simulink model "mfordmodel_v1"  (R2023a)
settings: Solver=ode45  StartTime=0.0  StopTime=10.0  RelTol=1e-3  EnableMultiTasking=on
undefined symbols (not defined in the file): ABV_RATIO_SW, AC_OFF_DLY, ACLOD, AUTO_TRNS_SW, BRAKE_DNDT_X, BZZRPM, BZZRPM_ALT, BZZTM, BZZTM_ALT, CMD_LITOFF, CMD_STABLE, CO_ST_ECT__A, COOL_BASE, DAS_BKDLY_A, DAS_CNT, DAS_CTDLY, DAS_LC_SW__A, DASCLP_5INH, DASCTL, DASMHYST, DASMPH, DEBYCP, DES_BASE, DPNEU_MUL, DSDRPM_DN_TC, DSDRPM_OFF, DSDRPM_UP_TC, EDF_DELAY, EDFHP, ETC_CL_TP, ETC_HP, GR_CM_CREEP, HCAM_ACT_CLP, HEDFHP, HEDFRPM, HICAM_PS, IAC_CAL_SW, IAC_ER_TM1, IAC_ER_TM2, IAC_ER_TM4, IAC_HI_LIM__A, IAC_ISFL_OBD, IAC_KAM_SW, IAC_LO_LIM__A, IAC_MON_TM, IAC_OT_REQ, IAC_RUN_TM, IAC_TP_OBD, IAC_TR_DAS, IAC_TST_DC, ID_DAS__A, ID_NOVS__A, IDVS_CH__A, IDVS_SL__A, IPSI_SW, IPSIDLY, IS_DRBASE__A, IS_DRBASE_A__A, IS_NUBASE__A, IS_NUBASE_A__A ... (+35)
libraries: simulink x2
(part 10 of 12)

== system mfordmodel_v1/iac_v04_001_001/normal_mode/activate_normal_mode/normal_mode_fault_codes/iac_er_tmr1/Time Calculator/timer_calculation/VAR SATURATION ==
  note: IF INPUT >= MAX THEN SWITHMAX ON
  note: IF INPUT <= MIN THEN SWITCH MIN ON
  MAX : Inport
  INPUT : Inport  Port=2
  MIN : Inport  Port=3
  From : From
  From1 : From
  Goto : Goto
  Logical Operator : Logic  Operator=OR
  Relational Operator : RelationalOperator
  Relational Operator1 : RelationalOperator  Operator=<=
  Switch : Switch  Threshold=0.5
  Switch2 : Switch  Threshold=0.5
  SwitchMAX : Switch  Threshold=0.5
  OUTPUT : Outport
  LIMIT_FLAG : Outport  Port=2
  wires:
  Logical Operator/1 -> LIMIT_FLAG/1
  Relational Operator1/1 -> Logical Operator/2, Switch/2
  Relational Operator/1 -> Logical Operator/1, Switch2/2, SwitchMAX/2
  MAX/1 -> Relational Operator/2, SwitchMAX/1
  SwitchMAX/1 -> Switch2/1
  Switch2/1 -> OUTPUT/1
  INPUT/1 -> Relational Operator/1, Relational Operator1/1, Goto/1
  From/1 -> Switch/3
  From1/1 -> SwitchMAX/3
  Switch/1 -> Switch2/3
  MIN/1 -> Relational Operator1/2, Switch/1

== system mfordmodel_v1/iac_v04_001_001/normal_mode/activate_normal_mode/normal_mode_fault_codes/iac_er_tmr2/Time Calculator/timer_calculation/VAR SATURATION ==
  note: IF INPUT >= MAX THEN SWITHMAX ON
  note: IF INPUT <= MIN THEN SWITCH MIN ON
  MAX : Inport
  INPUT : Inport  Port=2
  MIN : Inport  Port=3
  From : From
  From1 : From
  Goto : Goto
  Logical Operator : Logic  Operator=OR
  Relational Operator : RelationalOperator
  Relational Operator1 : RelationalOperator  Operator=<=
  Switch : Switch  Threshold=0.5
  Switch2 : Switch  Threshold=0.5
  SwitchMAX : Switch  Threshold=0.5
  OUTPUT : Outport
  LIMIT_FLAG : Outport  Port=2
  wires:
  Logical Operator/1 -> LIMIT_FLAG/1
  Relational Operator1/1 -> Logical Operator/2, Switch/2
  Relational Operator/1 -> Logical Operator/1, Switch2/2, SwitchMAX/2
  MAX/1 -> Relational Operator/2, SwitchMAX/1
  SwitchMAX/1 -> Switch2/1
  Switch2/1 -> OUTPUT/1
  INPUT/1 -> Relational Operator/1, Relational Operator1/1, Goto/1
  From/1 -> Switch/3
  From1/1 -> SwitchMAX/3
  Switch/1 -> Switch2/3
  MIN/1 -> Relational Operator1/2, Switch/1

== system mfordmodel_v1/iac_v04_001_001/normal_mode/activate_normal_mode/normal_mode_fault_codes/iac_mon_tmr/Time Calculator/timer_calculation/VAR SATURATION ==
  note: IF INPUT >= MAX THEN SWITHMAX ON
  note: IF INPUT <= MIN THEN SWITCH MIN ON
  MAX : Inport
  INPUT : Inport  Port=2
  MIN : Inport  Port=3
  From : From
  From1 : From
  Goto : Goto
  Logical Operator : Logic  Operator=OR
  Relational Operator : RelationalOperator
  Relational Operator1 : RelationalOperator  Operator=<=
  Switch : Switch  Threshold=0.5
  Switch2 : Switch  Threshold=0.5
  SwitchMAX : Switch  Threshold=0.5
  OUTPUT : Outport
  LIMIT_FLAG : Outport  Port=2
  wires:
  Logical Operator/1 -> LIMIT_FLAG/1
  Relational Operator1/1 -> Logical Operator/2, Switch/2
  Relational Operator/1 -> Logical Operator/1, Switch2/2, SwitchMAX/2
  MAX/1 -> Relational Operator/2, SwitchMAX/1
  SwitchMAX/1 -> Switch2/1
  Switch2/1 -> OUTPUT/1
  INPUT/1 -> Relational Operator/1, Relational Operator1/1, Goto/1
  From/1 -> Switch/3
  From1/1 -> SwitchMAX/3
  Switch/1 -> Switch2/3
  MIN/1 -> Relational Operator1/2, Switch/1

== system mfordmodel_v1/iac_v04_001_001/normal_mode/iscflg_module/dashpot/TIMER/Time Calculator/timer_calculation/VAR SATURATION ==
  note: IF INPUT >= MAX THEN SWITHMAX ON
  note: IF INPUT <= MIN THEN SWITCH MIN ON
  MAX : Inport
  INPUT : Inport  Port=2
  MIN : Inport  Port=3
  From : From
  From1 : From
  Goto : Goto
  Logical Operator : Logic  Operator=OR
  Relational Operator : RelationalOperator
  Relational Operator1 : RelationalOperator  Operator=<=
  Switch : Switch  Threshold=0.5
  Switch2 : Switch  Threshold=0.5
  SwitchMAX : Switch  Threshold=0.5
  OUTPUT : Outport
  LIMIT_FLAG : Outport  Port=2
  wires:
  Logical Operator/1 -> LIMIT_FLAG/1
  Relational Operator1/1 -> Logical Operator/2, Switch/2
  Relational Operator/1 -> Logical Operator/1, Switch2/2, SwitchMAX/2
  MAX/1 -> Relational Operator/2, SwitchMAX/1
  SwitchMAX/1 -> Switch2/1
  Switch2/1 -> OUTPUT/1
  INPUT/1 -> Relational Operator/1, Relational Operator1/1, Goto/1
  From/1 -> Switch/3
  From1/1 -> SwitchMAX/3
  Switch/1 -> Switch2/3
  MIN/1 -> Relational Operator1/2, Switch/1

== system mfordmodel_v1/iac_v04_001_001/normal_mode/iscflg_module/iscflg_modes/1/Time Calculator/timer_calculation/VAR SATURATION ==
  note: IF INPUT >= MAX THEN SWITHMAX ON
  note: IF INPUT <= MIN THEN SWITCH MIN ON
  MAX : Inport
  INPUT : Inport  Port=2
  MIN : Inport  Port=3
  From : From
  From1 : From
  Goto : Goto
  Logical Operator : Logic  Operator=OR
  Relational Operator : RelationalOperator
  Relational Operator1 : RelationalOperator  Operator=<=
  Switch : Switch  Threshold=0.5
  Switch2 : Switch  Threshold=0.5
  SwitchMAX : Switch  Threshold=0.5
  OUTPUT : Outport
  LIMIT_FLAG : Outport  Port=2
  wires:
  Logical Operator/1 -> LIMIT_FLAG/1
  Relational Operator1/1 -> Logical Operator/2, Switch/2
  Relational Operator/1 -> Logical Operator/1, Switch2/2, SwitchMAX/2
  MAX/1 -> Relational Operator/2, SwitchMAX/1
  SwitchMAX/1 -> Switch2/1
  Switch2/1 -> OUTPUT/1
  INPUT/1 -> Relational Operator/1, Relational Operator1/1, Goto/1
  From/1 -> Switch/3
  From1/1 -> SwitchMAX/3
  Switch/1 -> Switch2/3
  MIN/1 -> Relational Operator1/2, Switch/1

== system mfordmodel_v1/iac_v04_001_001/normal_mode/iscflg_module/iscflg_modes/2/Time Calculator/timer_calculation/VAR SATURATION ==
  note: IF INPUT >= MAX THEN SWITHMAX ON
  note: IF INPUT <= MIN THEN SWITCH MIN ON
  MAX : Inport
  INPUT : Inport  Port=2
  MIN : Inport  Port=3
  From : From
  From1 : From
  Goto : Goto
  Logical Operator : Logic  Operator=OR
  Relational Operator : RelationalOperator
  Relational Operator1 : RelationalOperator  Operator=<=
  Switch : Switch  Threshold=0.5
  Switch2 : Switch  Threshold=0.5
  SwitchMAX : Switch  Threshold=0.5
  OUTPUT : Outport
  LIMIT_FLAG : Outport  Port=2
  wires:
  Logical Operator/1 -> LIMIT_FLAG/1
  Relational Operator1/1 -> Logical Operator/2, Switch/2
  Relational Operator/1 -> Logical Operator/1, Switch2/2, SwitchMAX/2
  MAX/1 -> Relational Operator/2, SwitchMAX/1
  SwitchMAX/1 -> Switch2/1
  Switch2/1 -> OUTPUT/1
  INPUT/1 -> Relational Operator/1, Relational Operator1/1, Goto/1
  From/1 -> Switch/3
  From1/1 -> SwitchMAX/3
  Switch/1 -> Switch2/3
  MIN/1 -> Relational Operator1/2, Switch/1

== stateflow chart mfordmodel_v1/iac_v04_001_001/normal_mode/iscflg_module/iscflg_modes/activate_iscflg_mode_ctl ==
  (default) -> (junction 17) : trig_activate_iscflg_mode
  (junction 17) -> (junction 25) [order 1] : [ iscflg == ISCFLG_DASHPOT ]
      | {
      | trig_activate_daspot_mode;
      | id_mode = 0;
      | }
  (junction 17) -> (junction 18) [order 2]
  (junction 18) -> (junction 25) [order 1] : [ iscflg ==...
      |     ISCFLG_DASHPOT_PREPOSITION ]
      | {
      | trig_preposition;
      | id_mode = 0;
      | }
  (junction 18) -> (junction 19) [order 2]
  (junction 19) -> (junction 22) [order 1] : [ (iscflg ==...
      |     ISCFLG_RPM_CTRL_MODE) ...
      |  ||  (iscflg ==...
      |      ISCFLG_RPM_CTRL_NO_KAM_LEARN_MODE) ]
  (junction 19) -> (junction 20) [order 2]
  (junction 20) -> (junction 25) [order 2] : /* default: This branch
      |    should never be taken. */
  (junction 20) -> (junction 21) [order 1] : [ iscflg ==...
      |     ISCFLG_IDLE_DRIVE_MODE ]
  (junction 21) -> (junction 24) [order 1] : [ last_iscflg_tmp != iscflg ]
      | {
      | ml_idrv_init_flg = 1;
      | }
  (junction 22) -> (junction 23) [order 1] : [ last_iscflg_tmp < ISCFLG_RPM_CTRL_MODE ]
      | {
      | ml_irpm_init_flg = 1;
      | }
  (junction 21) -> (junction 24) [order 2] : {
      | ml_idrv_init_flg = 0;
      | }
  (junction 22) -> (junction 23) [order 2] : {
      | ml_irpm_init_flg = 0;
      | }
  (junction 23) -> (junction 25) : {
      | trig_idle_rpm_controller;
      | daspot = 0.0;
      | id_mode = 0;
      | }
  (junction 24) -> (junction 25) : {
      | trig_idle_drive_rpm_controller;
      | daspot = 0.0;
      | id_mode = 1;
      | }
  (junction 25) -> (junction 26) : {
      | last_iscflg_tmp = iscflg;
      | }
  data: last_iscflg_tmp local int8 size=1 =-1; ISCFLG_DASHPOT constant int8 size=1 =-1; ISCFLG_IDLE_DRIVE_MODE constant int8 size=1 =-2; ISCFLG_DASHPOT_PREPOSITION constant int8 size=1; ISCFLG_RPM_CTRL_MODE constant int8 size=1 =1; iscflg input int8 size=1; ml_idrv_init_flg output boolean size=1; ml_irpm_init_flg output boolean size=1; ISCFLG_RPM_CTRL_NO_KAM_LEARN_MODE constant int8 size=1 =2; daspot output single size=1; id_mode output boolean size=1
  events: trig_activate_daspot_mode output FUNCTION_CALL_EVENT; trig_activate_iscflg_mode input FUNCTION_CALL_EVENT; trig_preposition output FUNCTION_CALL_EVENT; trig_idle_rpm_controller output FUNCTION_CALL_EVENT; trig_idle_drive_rpm_controller output FUNCTION_CALL_EVENT

== stateflow chart mfordmodel_v1/iac_v04_001_001/normal_mode/activate_normal_mode/activate_normal_mode_ctl ==
  (default) -> (junction 9)
  (junction 9) -> (junction 11) [order 1] : [ vspd >= (DASMPH + DASMHYST) ]
      | {
      | flg_dasmnq = 1;
      | }
  (junction 9) -> (junction 10) [order 2]
  (junction 10) -> (junction 11) [order 2]
  (junction 10) -> (junction 11) [order 1] : [ vspd < DASMPH ]
      | {
      | flg_dasmnq = 0;
      | }
  (junction 11) -> (junction 12) [order 1] : [ tp > dstpbr ]
      | {
      | ml_tc_sw = 1;
      | }
  (junction 11) -> (junction 12) [order 2] : {
      | ml_tc_sw = 2;
      | }
  (junction 12) -> (junction 13) : {
      | do_dstpbr_calc;
      | trig_iscflg_modes ;
      | trig_activate_feedforward ;
      | trig_activate_kam ;
      | trig_ipsibr_clipping ;
      | trig_output_flow_calc ;
      | trig_normal_mode_fault_codes ;
      | }
  data: vspd input double size=1; ml_tc_sw output uint8 size=1; tp input double size=1; dstpbr input double size=1; DASMPH parameter double size=1; DASMHYST parameter double size=1; flg_dasmnq output boolean size=1
  events: trig_activate_normal_mode input FUNCTION_CALL_EVENT; trig_iscflg_modes output FUNCTION_CALL_EVENT; trig_activate_feedforward output FUNCTION_CALL_EVENT; trig_activate_kam output FUNCTION_CALL_EVENT; trig_ipsibr_clipping output FUNCTION_CALL_EVENT; trig_output_flow_calc output FUNCTION_CALL_EVENT; trig_normal_mode_fault_codes output FUNCTION_CALL_EVENT; do_dstpbr_calc output FUNCTION_CALL_EVENT

== stateflow chart mfordmodel_v1/iac_v04_001_001/normal_mode/iscflg_module/iscflg_modes/determine_iscflg_mode_ctl ==
  state normal_mode_reset [parallel]
    settings: executionOrder=1
    (default) -> (junction 63) : trig_normal_reset
    normal_mode_reset -> (junction 63) : trig_normal_reset
    (junction 63) -> (junction 68) : {
        | nlast = 0.0;
        | trig_settmr_reset;
        | }
  state transmission_state [parallel]
    settings: executionOrder=2
    transmission_state -> (junction 62) : trig
    (default) -> (junction 62) : trig
    (junction 62) -> (junction 67) [order 2] : {
        | trans_ok_tmp = 0;
        | }
    (junction 62) -> (junction 67) [order 1] : [ ( TRLOAD != 3 )...
        |   || ( dndsup == 0 ) ]
        | {
        | trans_ok_tmp = 1;
        | }
    (junction 67) -> (junction 72) [order 2] : {
        | id_trans_ok_tmp = 0;
        | }
    (junction 67) -> (junction 70) [order 1] : [ ( novs_mtx__A > ID_NOVS__A)...
        |  && ( novs_mtx__A < 254.0 )...
        |  && ( ndsflg == 1) ]
    (junction 70) -> (junction 72) : [ ( TRLOAD == 3 )...
        |  || ( TRLOAD == 2 ) ]
        | {
        | id_trans_ok_tmp = 1;
        | }
  state vehicle_speed_check [parallel]
    settings: executionOrder=3
    vehicle_speed_check -> (junction 64) : trig
    (default) -> (junction 64) : trig
    (junction 64) -> (junction 71) [order 1] : [ vspd < IDVS_SL__A ]
        | {
        | id_lo_spd = 1;
        | }
    (junction 64) -> (junction 66) [order 2]
    (junction 66) -> (junction 71) [order 1] : [ vspd > IDVS_CH__A ]
        | {
        | id_lo_spd = 0;
        | }
    (junction 66) -> (junction 71) [order 2]
    (junction 71) -> (junction 74) [order 1] : [ vspd <= MINMPH ]
        | {
        | lo_spd_tmp = 1;
        | }
    (junction 71) -> (junction 74) [order 2] : {
        | lo_spd_tmp = 0;
        | }
  state bleed_level_check [parallel]
    settings: executionOrder=4
    bleed_level_check -> (junction 65) : trig
    (default) -> (junction 65) : trig
    (junction 65) -> (junction 69) [order 2] : {
        | id_das_low_tmp = 0;
        | }
    (junction 65) -> (junction 69) [order 1] : [   ( idle_ppm <= ID_DAS__A )...
        |  || ( iscflg == ISCFLG_IDLE_DRIVE_MODE ) ]
        | {
        | id_das_low_tmp = 1;
        | }
    (junction 69) -> (junction 73) [order 2] : {
        | das_low_tmp = 0;
        | trig_settmr_reset;
        | }
    (junction 69) -> (junction 73) [order 1] : [   (     ( idle_ppm <= DASCTL )...
        |     && ( iscflg != ISCFLG_DASHPOT_PREPOSITION ) )...
        |  || ( iscflg >= ISCFLG_RPM_CTRL_MODE)  ]
        | {
        | das_low_tmp = 1;
        | trig_settmr_update;
        | }
    (junction 73) -> (junction 75) [order 2] : {
        | manifold_stbl_tmp = 0;
        | }
    (junction 73) -> (junction 75) [order 1] : [  settmr > SETLNG_TM ]
        | {
        | manifold_stbl_tmp = 1;
        | }
  state decel_check [parallel]
    settings: executionOrder=5
    decel_check -> (junction 76) : trig
    (default) -> (junction 76) : trig
    (junction 76) -> (junction 78) [order 2] : {
        | aclod_tmp = 0.0;
        | }
    (junction 76) -> (junction 78) [order 1] : [ accflg == 1 ]
        | {
        | aclod_tmp = ACLOD;
        | }
    (junction 78) -> (junction 88) [order 1] : [ iscflg >=...
        |    ISCFLG_RPM_CTRL_MODE ]
        | {
        | lockout_tmp = 1;
        | }
    (junction 78) -> (junction 79) [order 2]
    (junction 79) -> (junction 80) [order 2]
    (junction 79) -> (junction 88) [order 1] : [ isctmr < ISCTM ]
        | {
        | lockout_tmp = 0;
        | }
    (junction 80) -> (junction 81) [order 2]
    (junction 80) -> (junction 88) [order 1] : [ fabs( engine_speed - nlast ) > NDIF ]
        | {
        | lockout_tmp = 0;
        | nlast = engine_speed;
        | trig_isctmr_reset;
        | }
    (junction 81) -> (junction 83) [order 2]
    (junction 81) -> (junction 88) [order 1] : [ ( TRLOAD >= 2 )...
        |  && ( dndsup == 0 ) ]
        | {
        | lockout_tmp = 1;
        | }
    (junction 83) -> (junction 88) [order 2] : {
        | lockout_tmp = 1;
        | }
    (junction 83) -> (junction 88) [order 1] : [ load <...
        |   ( LOWLOD + aclod_tmp) ]
        | {
        | lockout_tmp = 0;
        | }
    (junction 88) -> (junction 89) [order 2] : {
        | trig_isctmr_update;
        | }
    (junction 88) -> (junction 89) [order 1] : [ apt >= 0 ]
        | {
        | trig_isctmr_reset;
        | nlast = engine_speed;
        | }
  state determine_iscflg_mode [parallel]
    settings: executionOrder=6
    determine_iscflg_mode -> (junction 77) : trig_determine_iscflg_mode
    (default) -> (junction 77) : trig_determine_iscflg_mode
    (junction 77) -> (junction 82) : {
        | iscflg = iscflg_in; /* For Matlab Only */
        | bleed_level_check.trig;
        | vehicle_speed_check.trig;
        | decel_check.trig;
        | transmission_state.trig;
        | }
    (junction 82) -> (junction 84) [order 2] : {
        | delay_rpm_ctrl_tmp = 0;
        | }
    (junction 82) -> (junction 84) [order 1] : [ runuptmr < IPSIDLY ]
        | {
        | delay_rpm_ctrl_tmp = 1;
        | }
    (junction 85) -> (junction 86) [order 2]
    (junction 84) -> (junction 90) [order 1] : [ apt != CLOSED_THROTTLE ]
        | {
        | iscflg =...
        |    ISCFLG_DASHPOT_PREPOSITION;
        | }
    (junction 84) -> (junction 85) [order 2]
    (junction 85) -> (junction 90) [order 1] : [ ( das_low_tmp == 1 )...
        |  && ( trans_ok_tmp == 1 )...
        |  && ( engine_speed < (dsdrpm + RPMCTL) )...
        |  && ( delay_rpm_ctrl_tmp == 0 )...
        |  && ( manifold_stbl_tmp == 1 )...
        |  && ( lo_spd_tmp ==1 ) ]
        | {
        | iscflg =...
        |    ISCFLG_RPM_CTRL_MODE;
        | }
    (junction 86) -> (junction 87) [order 2]
    (junction 86) -> (junction 90) [order 1] : [ ( das_low_tmp == 1 )...
        |  && ( trans_ok_tmp == 1 )...
        |  && ( lockout_tmp == 1 )...
        |  && ( delay_rpm_ctrl_tmp == 0 )...
        |  && ( manifold_stbl_tmp == 1 )...
        |  && ( lo_spd_tmp ==1 ) ]
        | {
        | iscflg =...
        |    ISCFLG_RPM_CTRL_NO_KAM_LEARN_MODE;
        | }
    (junction 87) -> (junction 90) [order 2] : {
        | iscflg = ISCFLG_DASHPOT;
        | }
    (junction 87) -> (junction 90) [order 1] : [ ( id_das_low_tmp == 1)...
        |  && ( id_trans_ok_tmp == 1 )...
        |  && (id_lo_spd == 1 ) ]
        | {
        | iscflg =...
        |   ISCFLG_IDLE_DRIVE_MODE;
        | }
  data: engine_speed input double size=1; vspd input double size=1; load input double size=1; dndsup input boolean size=1; apt input int8 size=1; iscflg output int8 size=1; ACLOD parameter double size=1; DASCTL parameter double size=1; IDVS_CH__A parameter double size=1; IDVS_SL__A parameter double size=1; ID_DAS__A parameter double size=1; ID_NOVS__A parameter double size=1; ISCTM parameter double size=1; LOWLOD parameter double size=1; MINMPH parameter double size=1; SETLNG_TM parameter double size=1; TRLOAD parameter uint8 size=1; NDIF parameter double size=1; DASMHYST parameter double size=1; DASMPH parameter double size=1; CLOSED_THROTTLE constant int8 size=1 =-1; runuptmr input double size=1; ISCFLG_DASHPOT_PREPOSITION constant uint8 size=1; IPSIDLY parameter double size=1; id_das_low_tmp local boolean size=1; id_lo_spd local boolean size=1; lo_spd_tmp local boolean size=1; delay_rpm_ctrl_tmp local boolean size=1; lockout_tmp local boolean size=1; aclod_tmp local double size=1; accflg input boolean size=1; trans_ok_tmp local boolean size=1; id_trans_ok_tmp local boolean size=1; ISCFLG_RPM_CTRL_MODE constant int8 size=1 =1; ISCFLG_IDLE_DRIVE_MODE constant int8 size=1 =-2; ISCFLG_DASHPOT constant int8 size=1 =-1; manifold_stbl_tmp local boolean size=1; idle_ppm input double size=1; ndsflg input boolean size=1; novs_mtx__A input double size=1; iscflg_in input uint8 size=1; dsdrpm input double size=1; isctmr input double size=1; settmr input double size=1; das_low_tmp local boolean size=1; ml_normal_init local uint8 size=1; nlast local double size=1; ISCFLG_RPM_CTRL_NO_KAM_LEARN_MODE constant int8 size=1 =2; RPMCTL parameter double size=1
  events: trig local EITHER_EDGE_EVENT; trig local EITHER_EDGE_EVENT; trig local EITHER_EDGE_EVENT; trig local EITHER_EDGE_EVENT; trig local EITHER_EDGE_EVENT; trig_determine_iscflg_mode input FUNCTION_CALL_EVENT; trig_isctmr_reset output FUNCTION_CALL_EVENT; trig_isctmr_update output FUNCTION_CALL_EVENT; trig_settmr_reset output FUNCTION_CALL_EVENT; trig_settmr_update output FUNCTION_CALL_EVENT; trig_normal_reset input FUNCTION_CALL_EVENT

== stateflow chart mfordmodel_v1/iac_v04_001_001/normal_mode/activate_normal_mode/ipsibr_clipping/ipsibr_clipping_ctl ==
  (default) -> (junction 14)
  (junction 14) -> (junction 17) [order 1] : [ ml_normal_init == 1 ]
  (junction 14) -> (junction 15) [order 2]
  (junction 15) -> (junction 16) [order 2] : {
      | ml_min_clip = 2;
      | }
  (junction 15) -> (junction 16) [order 1] : [ ( isflag != islast )...
      |   || ( ctptfg == 1 )   ]
      | {
      | ml_min_clip = 1;
      | }
  (junction 16) -> (junction 17) [order 1] : [      ( IPSI_SW == 1 )...
      |  && ( iscflg <= ISCFLG_DASHPOT_PREPOSITION      )       ]
      | {
      | ml_max_clip = 1;
      | }
  (junction 16) -> (junction 17) [order 2] : {
      | ml_max_clip = 2;
      | }
  (junction 17) -> (junction 18) [order 1] : [ (PRG_FLOW_SW == 0)...
      |   || (flow_running == 0) ]
  (junction 17) -> (junction 19) [order 2]
  (junction 18) -> (junction 20) [order 1] : [      (ipsibr < 0.0)...
      |  && (lpcomp_ena == 1)...
      |  && (pcomp_ena == 0)...
      |  && (PUR_ENA_SW == 1) ]
      | {
      |  ml_limit_sw = 2;
      | }
  (junction 18) -> (junction 19) [order 2]
  (junction 19) -> (junction 20) : {
      | ml_limit_sw = 1;
      |  }
  (junction 20) -> (junction 21) : {
      | lpcomp_ena = pcomp_ena;
      | do_ipsibr_clip ;
      | }
  data: isflag input uint8 size=1; islast input uint8 size=1; ctptfg input boolean size=1; iscflg input boolean size=1; ml_max_clip output uint8 size=1 =1; ml_min_clip output uint8 size=1 =1; IPSI_SW parameter boolean size=1; ISCFLG_DASHPOT_PREPOSITION constant uint8 size=1; ml_normal_init input uint8 size=1; ipsibr input single size=1; flow_running input boolean size=1; pcomp_ena input boolean size=1; PUR_ENA_SW parameter boolean size=1; PRG_FLOW_SW parameter boolean size=1; lpcomp_ena local boolean size=1; ml_limit_sw output int8 size=1 =1
  events: trig_ipsibr_clipping input FUNCTION_CALL_EVENT; do_ipsibr_clip output FUNCTION_CALL_EVENT

== stateflow chart mfordmodel_v1/iac_v04_001_001/normal_mode/activate_normal_mode/normal_mode_fault_codes/normal_mode_fault_codes_ctl ==
  (default) -> (junction 27)
  (junction 27) -> (junction 40) [order 2] : { trig_er_tmr1_reset;
      |    trig_er_tmr2_reset; }
  (junction 27) -> (junction 28) [order 1] : [ ml_normal_init == 2 ]
      | { iac_err1 = 0;
      |   iac_err2 = 0;
      |   iac_tst_run = 1; }
  (junction 28) -> (junction 29) [order 1] : [     (p0171malf == 0)...
      |  && (p0172malf == 0)...
      |  && (p0174malf == 0)...
      |  && (p0175malf == 0)  ]
      | { iac_fuel_ok = 1; }
  (junction 28) -> (junction 29) [order 2] : { iac_fuel_ok = 0; }
  (junction 29) -> (junction 32) [order 1] : [ (iscflg <= ISCFLG_DASHPOT_PREPOSITION )...
      |     || (vspd > 0.0 )...
      |     || (runuptmr < IPSIDLY )...
      |     || (uspd_run_tmr < IAC_RUN_TM  )...
      |     || (isflag > IAC_ISFL_OBD )...
      |     || (ect < CO_ST_ECT__A  )...
      |     || (V_IAC_TST == 0 )...
      |     || (ffg_ect == 1 )...
      |     || (vsfmflg == 1 )...
      |     || (ffg_tp ==1 )...
      |     || (tp_rel > IAC_TP_OBD )...
      |     || (powsfg ==1 )...
      |     || (obdii_reset == 1 )...
      |     || (iac_fuel_ok == 0 )...
      |     || (pto_active == 1 )  ]
  (junction 29) -> (junction 32) [order 2] : [   ( ccm_tst_ena == 0)...
      |   && (er_status != ISC_LO_CHECK) ]
  (junction 29) -> (junction 30) [order 3]
  (junction 30) -> (junction 33) [order 1] : [     (pdl_error == 0 )...
      | && (rpmerr_a < IAC_HI_LIM__A)...
      | && (iac_at_lolm == 1 )   ]
      | { iac_err1 =1; }
  (junction 30) -> (junction 31) [order 2]
  (junction 31) -> (junction 33) [order 2]
  (junction 31) -> (junction 33) [order 1] : [      (rpmerr_a >= IAC_LO_LIM__A )...
      |  && (  (iac_at_hilm ==1   )...
      |         || (iac_fb_satx  )  )  ]
      | { iac_err2 = 1; }
  (junction 32) -> (junction 33) : { iac_tst_run = 0; }
  (junction 33) -> (junction 35) [order 1] : [ iac_err1 == 0 ]
      | { trig_er_tmr1_reset; }
  (junction 33) -> (junction 34) [order 2]
  (junction 34) -> (junction 35) [order 1] : [  ( iac_err1 == 1 )...
      |  && ( iac_er_tmr1 > IAC_ER_TM1 )   ]
      | { trig_malfunction_p1506;
      |    trig_er_tmr1_reset;  }
  (junction 34) -> (junction 35) [order 2] : { trig_clear_malf_p1506 ;
      |   trig_er_tmr1_update ; }
  (junction 35) -> (junction 37) [order 1] : [ iac_err2 == 0 ]
      | { trig_er_tmr2_reset; }
  (junction 35) -> (junction 36) [order 2]
  (junction 36) -> (junction 37) [order 1] : [  ( iac_err2 == 1 )...
      |  && ( iac_er_tmr2 > IAC_ER_TM2 )   ]
      | { trig_malfunction_p1507;
      |    trig_er_tmr2_reset;  }
  (junction 36) -> (junction 37) [order 2] : { trig_clear_malf_p1507 ;
      |   trig_er_tmr2_update ; }
  (junction 37) -> (junction 38) [order 2]
  (junction 37) -> (junction 38) [order 1] : [(iac_mon_tmr > IAC_MON_TM)...
      |  || (V_IAC_TST == 0) ]
      | { ccm_iac_mon = 1; }
  (junction 38) -> (junction 39) [order 1] : [  iac_tst_run == 0  ]
      | { trig_mon_tmr_reset; }
  (junction 38) -> (junction 39) [order 2] : { trig_mon_tmr_update; }
  (junction 39) -> (junction 40) : { do_update_pids; }
  data: ccm_iac_mon output boolean size=1; iac_fuel_ok local boolean size=1; iac_err1 local boolean size=1; iac_err2 local boolean size=1; iac_tst_run local boolean size=1; runuptmr input double size=1; rpmerr_a input double size=1; iac_at_lolm input double size=1; iac_at_hilm input double size=1; iac_fb_satx input double size=1; uspd_run_tmr input double size=1; apt input double size=1; vspd input double size=1; ect input double size=1; tp_rel input double size=1; powsfg input double size=1; ccm_tst_ena input double size=1; er_status input double size=1; ffg_ect input double size=1; vsfmflg input double size=1; ffg_tp input double size=1; obdii_reset input double size=1; pto_active input double size=1; pdl_error input boolean size=1; p0171malf input boolean size=1; p0172malf input boolean size=1; p0174malf input boolean size=1; p0175malf input boolean size=1; isflag input double size=1; iscflg input double size=1; ml_normal_init input boolean size=1; iac_er_tmr1 input double size=1; iac_er_tmr2 input double size=1; iac_mon_tmr input double size=1; CO_ST_ECT__A parameter double size=1; IAC_ER_TM1 parameter double size=1; IAC_ER_TM2 parameter double size=1; IAC_HI_LIM__A parameter double size=1; IAC_ISFL_OBD parameter double size=1; IAC_LO_LIM__A parameter double size=1; IAC_MON_TM parameter double size=1; IAC_RUN_TM parameter double size=1; IAC_TP_OBD parameter double size=1; IPSIDLY parameter double size=1; ISC_LO_CHECK parameter double size=1; V_IAC_TST parameter double size=1; ISCFLG_DASHPOT_PREPOSITION constant uint8 size=1
  events: do_update_pids output FUNCTION_CALL_EVENT; trig_malfunction_p1506 output FUNCTION_CALL_EVENT; trig_clear_malf_p1506 output FUNCTION_CALL_EVENT; trig_malfunction_p1507 output FUNCTION_CALL_EVENT; trig_clear_malf_p1507 output FUNCTION_CALL_EVENT; trig_er_tmr1_update output FUNCTION_CALL_EVENT; trig_er_tmr1_reset output FUNCTION_CALL_EVENT; trig_er_tmr2_update output FUNCTION_CALL_EVENT; trig_er_tmr2_reset output FUNCTION_CALL_EVENT; trig_normal_mode_fault_codes input FUNCTION_CALL_EVENT; trig_mon_tmr_update output FUNCTION_CALL_EVENT; trig_mon_tmr_reset output FUNCTION_CALL_EVENT

== stateflow chart mfordmodel_v1/iac_v04_001_001/normal_mode/activate_normal_mode/output_flow_calc/output_flow_calc_ctl ==
  (default) -> (junction 15) : {
      | do_tr_dsdrpm_calc ;
      | }
  (junction 15) -> (junction 16) [order 1] : [     (TR_DSDRPM_SW == 1)...
      |    && (ml_tr_dsdrpm_calc > 0.0)     ]
      | {
      | ml_tr_dsdrpm_sw = 1 ;
      | }
  (junction 15) -> (junction 16) [order 2] : {
      | ml_tr_dsdrpm_sw = 2 ;
      | }
  (junction 16) -> (junction 17) [order 2] : {
      |  ml_tr_das_sw = 1;
      | }
  (junction 16) -> (junction 17) [order 1] : [ IAC_TR_DAS == 1 ]
      | {
      |  ml_tr_das_sw = 2;
      | }
  (junction 17) -> (junction 18) [order 2] : {
      | ml_flowrate_sw = 1;
      | }
  (junction 17) -> (junction 18) [order 1] : [ IAC_CAL_SW == 1 ]
      | {
      |  ml_flowrate_sw = 2;
      | }
  (junction 18) -> (junction 19) [order 2] : {
      |  ml_ratio_sw = 1;
      | }
  (junction 18) -> (junction 19) [order 1] : [ ABV_RATIO_SW == 1 ]
      | {
      |  ml_ratio_sw = 2;
      | }
  (junction 19) -> (junction 20) : {
      | ml_isflag_sw = isflag + 1;
      | do_desmaf_calc ;
      | }
  (junction 20) -> (junction 21) [order 2] : {
      |  iac_at_lolm = 0;
      | }
  (junction 20) -> (junction 21) [order 1] : [ abv_flowrate <= DEBYCP ]
      | {
      |  iac_at_lolm = 1;
      | }
  (junction 21) -> (junction 22) [order 1] : [ abv_status & 0x02 ]
      | {
      |  iac_at_hilm = 1;
      | }
  (junction 21) -> (junction 22) [order 2] : {
      |  iac_at_hilm = 0;
      | }
  data: iac_at_lolm output double size=1; iac_at_hilm output double size=1; abv_status input int16 size=1; isflag input uint8 size=1; abv_flowrate input double size=1; ml_tr_dsdrpm_calc input double size=1; DEBYCP parameter double size=1; TR_DSDRPM_SW parameter double size=1; ml_tr_dsdrpm_sw output uint8 size=1; ml_flowrate_sw output uint8 size=1; ml_tr_das_sw output uint8 size=1; ml_ratio_sw output uint8 size=1; IAC_TR_DAS parameter boolean size=1; IAC_CAL_SW parameter boolean size=1; ABV_RATIO_SW parameter boolean size=1; ml_isflag_sw output uint8 size=1
  events: trig_output_flow_calc input FUNCTION_CALL_EVENT; do_desmaf_calc output FUNCTION_CALL_EVENT; do_tr_dsdrpm_calc output FUNCTION_CALL_EVENT

== stateflow chart mfordmodel_v1/iac_v04_001_001/normal_mode/iscflg_module/dashpot/daspot_shift_trans_calc_ctl ==
  state Note: [group]
    The parallel state "downshifts"must be placed at a
    higher priority than "upshifts".
  state downshifts [parallel]
    settings: executionOrder=1
    (default) -> (junction 103) : trig
    downshifts -> (junction 103) : trig
    (junction 103) -> (junction 104) [order 1] : [ (gr_old == 5 )...
        |   && (pdl <= 44 )...
        |   && (gr_cm == 4) ]
    (junction 104) -> (junction 109) : /* 5 - 4 Down Shift */
        | { das_ppm__A = ml_fn899;
        |   das_tc__A = TC_MAN54;
        |   flg_das = 1; }
    (junction 103) -> (junction 107) [order 2]
    (junction 107) -> (junction 108) [order 1] : [ (gr_old == 5)...
        |   && (pdl <= 23 )...
        |   && (gr_cm == 3) ]
    (junction 109) -> (junction 110)
    (junction 108) -> (junction 115) : { das_ppm__A = ml_fn899 * MAN_MULT53;
        |   das_tc__A = TC_MAN53;}
    (junction 110) -> (junction 116) : /* 5 - 3 Down Shift */
    (junction 107) -> (junction 117) [order 2]
    (junction 115) -> (junction 116)
    (junction 116) -> (junction 122) : /* 5 - 2 Down Shift */
    (junction 117) -> (junction 118) [order 1] : [ (gr_old == 5)...
        |   && (pdl <= 22 )...
        |   && (gr_cm == 2) ]
    (junction 118) -> (junction 123) : { das_ppm__A = ml_fn899 * MAN_MULT52;
        |   das_tc__A = TC_MAN52; }
    (junction 117) -> (junction 124) [order 2]
    (junction 123) -> (junction 122)
    (junction 122) -> (junction 131) : /* 4 - 3  Down Shift */
    (junction 124) -> (junction 125) [order 1] : [ (gr_old == 4)...
        |   && (pdl <= 23 )...
        |   && (gr_cm == 3) ]
    (junction 125) -> (junction 130) : { das_ppm__A = ml_fn899 * MAN_MULT43;
        |   das_tc__A = TC_MAN43__A;
        |   flg_das = 1; }
    (junction 124) -> (junction 132) [order 2]
    (junction 130) -> (junction 131)
    (junction 131) -> (junction 139) : /* 4 - 2  Down Shift */
    (junction 132) -> (junction 133) [order 1] : [ (gr_old == 4)...
        |   && (pdl <= 22 )...
        |   && (gr_cm == 2) ]
    (junction 133) -> (junction 138) : { das_ppm__A = ml_fn899 * MAN_MULT42__A;
        |   das_tc__A = TC_MAN42__A;
        |   flg_das = 1; }
    (junction 132) -> (junction 140) [order 2]
    (junction 138) -> (junction 139)
    (junction 139) -> (junction 147) : /* 4 - 1  Down Shift */
    (junction 140) -> (junction 141) [order 1] : [ (gr_old == 4)...
        |   && (pdl == 21 )...
        |   && (gr_cm == 1) ]
    (junction 141) -> (junction 146) : { das_ppm__A = ml_fn899 * MAN_MULT41;
        |   das_tc__A = TC_MAN41;
        |   flg_das = 1; }
    (junction 140) -> (junction 148) [order 2]
    (junction 146) -> (junction 147)
    (junction 147) -> (junction 155) : /* 3 - 2  Down Shift */
    (junction 148) -> (junction 149) [order 1] : [ (gr_old == 3)...
        |   && (pdl <= 22 )...
        |   && (gr_cm == 2) ]
    (junction 149) -> (junction 154) : { das_ppm__A = ml_fn899 * MAN_MULT32__A;
        |   das_tc__A = TC_MAN32__A;
        |   flg_das = 1; }
    (junction 148) -> (junction 156) [order 2]
    (junction 154) -> (junction 155)
    (junction 155) -> (junction 163) : /* 3 - 1  Down Shift */
    (junction 156) -> (junction 157) [order 1] : [ (gr_old == 3)...
        |   && (pdl == 21 )...
        |   && (gr_cm == 1) ]
    (junction 157) -> (junction 162) : { das_ppm__A = ml_fn899 * MAN_MULT31;
        |   das_tc__A = TC_MAN31;
        |   flg_das = 1; }
    (junction 156) -> (junction 164) [order 2]
    (junction 162) -> (junction 163)
    (junction 163) -> (junction 171) : /* 2 - 1  Down Shift */
    (junction 164) -> (junction 165) [order 1] : [ (gr_old == 2)...
        |   && (pdl == 21 )...
        |   && (gr_cm == 1) ]
    (junction 165) -> (junction 170) : { das_ppm__A = ml_fn899 * MAN_MULT21;
        |   das_tc__A = TC_MAN21;
        |   flg_das = 1; }
    (junction 164) -> (junction 172) [order 2] : /* ELSE */
        | { das_ppm__A = 0.0;
        |   das_tc__A = 0.0;
        |   ml_das_delay = 0.0;
        |   flg_das = 0; }
    (junction 170) -> (junction 171)
    (junction 171) -> (junction 173) : { ml_das_delay =...
        |     DLY_MAN_DN__A; }
    (junction 173) -> (junction 172)
  state upshifts [parallel]
    settings: executionOrder=2
    upshifts -> (junction 102)
    (default) -> (junction 102)
    (junction 102) -> (junction 105) : { do_function_calcs; }
    (junction 105) -> (junction 106) [order 1] : [ ( flg_sft_in == 0 )...
        |   && ( gr_cm == igr_ds) ]
    (junction 106) -> (junction 112)
    (junction 105) -> (junction 111) [order 2]
    (junction 111) -> (junction 112) [order 1] : [ apt != CLOSED_THROTTLE ]
    (junction 112) -> (junction 119) : { das_ppm__A = 0.0;
        |   das_tc__A = 0.0;
        |   ml_das_delay = 0.0;
        |   flg_das = 0; }
    (junction 111) -> (junction 113) [order 2]
    (junction 113) -> (junction 114) [order 1] : /* Shift in progress? */
        |     [ flg_das == 1 ]
    (junction 114) -> (junction 178)
    (junction 113) -> (junction 120) [order 2]
    (junction 119) -> (junction 127) : /* 1 - 2 Up Shiftt */
    (junction 120) -> (junction 121) [order 1] : [ (gr_cm_lst == 1)...
        |   && ( gr_cm == 2) ]
    (junction 121) -> (junction 126) : { das_ppm__A = ml_fnbo12;
        |   das_tc__A = TC_BO12__A;
        |   ml_das_delay = DLY_BO12__A;
        |   flg_das = 1; }
    (junction 120) -> (junction 128) [order 2]
    (junction 126) -> (junction 127)
    (junction 127) -> (junction 135) : /* 1 - 3 Up Shift */
    (junction 128) -> (junction 129) [order 1] : [ (gr_cm_lst == 1)...
        |   && (gr_cm == 3) ]
    (junction 129) -> (junction 134) : { das_ppm__A = ml_fnbo13;
        |   das_tc__A = TC_BO13__A;
        |   ml_das_delay = DLY_BO13__A;
        |   flg_das = 1; }
    (junction 128) -> (junction 136) [order 2]
    (junction 134) -> (junction 135)
    (junction 135) -> (junction 143) : /* 2 - 3 Up Shift */
    (junction 136) -> (junction 137) [order 1] : [ (gr_cm_lst == 2)...
        |   && (gr_cm == 3) ]
    (junction 137) -> (junction 142) : { das_ppm__A = ml_fnbo23;
        |   das_tc__A = TC_BO23__A;
        |   ml_das_delay = DLY_BO23__A;
        |   flg_das = 1; }
    (junction 136) -> (junction 144) [order 2]
    (junction 142) -> (junction 143)
    (junction 143) -> (junction 151) : /* 2 - 4 Up Shift */
    (junction 144) -> (junction 145) [order 1] : [ (gr_cm_lst == 2)...
        |    && (gr_cm == 4) ]
    (junction 145) -> (junction 150) : { das_ppm__A = ml_fnbo24;
        |   das_tc__A = TC_BO24__A;
        |   ml_das_delay = DLY_BO24;
        |   flg_das = 1; }
    (junction 144) -> (junction 152) [order 2]
    (junction 150) -> (junction 151)
    (junction 151) -> (junction 159) : /* 3 - 4 Up Shift*/
    (junction 152) -> (junction 153) [order 1] : [ (gr_cm_lst == 3)...
        |   && (gr_cm == 4) ]
    (junction 153) -> (junction 158) : { das_ppm__A = ml_fnbo34;
        |   das_tc__A = TC_BO34__A;
        |   ml_das_delay = DLY_BO34;
        |   flg_das = 1; }
    (junction 152) -> (junction 160) [order 2]
    (junction 158) -> (junction 159)
    (junction 159) -> (junction 167) : /* 3 - 5 Up Shift */
    (junction 160) -> (junction 161) [order 1] : [ (gr_cm_lst == 3)...
        |   && (gr_cm == 5) ]
    (junction 161) -> (junction 166) : { das_ppm__A = ml_fnbo35;
        |   das_tc__A = TC_BO35__A;
        |   ml_das_delay = DLY_BO35;
        |   flg_das = 1; }
    (junction 160) -> (junction 168) [order 2]
    (junction 166) -> (junction 167)
    (junction 167) -> (junction 176) : /* 4 - 5 Up Shift */
    (junction 168) -> (junction 169) [order 1] : [ (gr_cm_lst == 4)...
        |   && (gr_cm == 5) ]
    (junction 169) -> (junction 175) : { das_ppm__A = ml_fnbo45;
        |   das_tc__A = TC_BO45__A;
        |   ml_das_delay = DLY_BO45;
        |   flg_das = 1; }
    (junction 168) -> (junction 174) [order 2] : { downshifts.trig; }
    (junction 175) -> (junction 174)
    (junction 176) -> (junction 175)
    (junction 174) -> (junction 177) : { trig_rst_das_delay; }
    (junction 178) -> (junction 177)
  data: flg_das local boolean size=1; igr_ds input boolean size=1; flg_sft_in input boolean size=1; CLOSED_THROTTLE constant int8 size=1 =-1; gr_old input uint8 size=1; gr_cm input uint8 size=1; gr_cm_lst input uint8 size=1; pdl input uint8 size=1; das_ppm__A output single size=1; das_tc__A output single size=1; ml_das_delay output single size=1; TC_BO12__A constant single size=1; DLY_BO12__A constant single size=1; apt input int8 size=1; ml_fn899 input single size=1; ml_fnbo12 input single size=1; ml_fnbo13 input single size=1; ml_fnbo23 input single size=1; DLY_MAN_DN__A constant single size=1; ml_fnbo24 input single size=1; ml_fnbo34 input single size=1; ml_fnbo35 input single size=1; ml_fnbo45 input single size=1; TC_BO13__A constant single size=1; TC_BO23__A constant single size=1; TC_BO24__A constant single size=1; TC_BO34__A constant single size=1; TC_BO35__A constant single size=1; TC_BO45__A constant single size=1; TC_MAN54 constant single size=1; TC_MAN53 constant single size=1; TC_MAN52 constant single size=1; TC_MAN43__A constant single size=1; TC_MAN42__A constant single size=1; TC_MAN41 constant single size=1; TC_MAN32__A constant single size=1; TC_MAN31 constant single size=1; TC_MAN21 constant single size=1; DLY_BO13__A constant single size=1; DLY_BO23__A constant single size=1; DLY_BO24 constant single size=1; DLY_BO34 constant single size=1; DLY_BO35 constant single size=1; DLY_BO45 constant single size=1; MAN_MULT53 constant single size=1; MAN_MULT52 constant single size=1; MAN_MULT43 constant single size=1; MAN_MULT42__A constant single size=1; MAN_MULT41 constant single size=1; MAN_MULT32__A constant single size=1; MAN_MULT31 constant single size=1; MAN_MULT21 constant single size=1
  events: trig local EITHER_EDGE_EVENT; trig_daspot_shift_trans_calc input FUNCTION_CALL_EVENT; trig_rst_das_delay output FUNCTION_CALL_EVENT; do_function_calcs output FUNCTION_CALL_EVENT

== stateflow chart mfordmodel_v1/iac_v04_001_001/normal_mode/iscflg_module/iscflg_modes/iscflg_modes_ctl ==
  (default) -> (junction 4) : trig_iscflg_modes
  (junction 4) -> (junction 5) [order 2] : {
      | trig_normal_reset;
      | }
  (junction 4) -> (junction 5) [order 1] : [ ml_normal_init == 2 ]
      | {
      | trig_determine_iscflg_mode;
      | trig_activate_iscflg_mode;
      | }
  data: ml_normal_init input double size=1
  events: trig_iscflg_modes input FUNCTION_CALL_EVENT; trig_activate_iscflg_mode output FUNCTION_CALL_EVENT; trig_determine_iscflg_mode output FUNCTION_CALL_EVENT; trig_normal_reset output FUNCTION_CALL_EVENT

== stateflow chart mfordmodel_v1/iac_v04_001_001/iac_executive/fault_code_setting/fault_code_setting_ctl ==
  (default) -> (junction 10) : /*
      | SCCD IAC driver diagnostics:  The SCCD/DARC I/O chips provide
      | idle speed control valve (IAC) driver fault status (abv_status) to the
      | strategy. The states of over  current and under current are diagnosed.
      | PIDs are separately defined but  both faults will set the same OBDII
      | fault code (P1504). It is not possible to detect an over current condition
      | when ISCDTY is zero. The associated error timer is therefore frozen
      | when the ISC dutycycle is below a calibrateable level and the open
      | load/ground short fault  bit (IAC_NO_CUR) is not set.
      |
      |               abv_status:    BIT3 (0x08) = No current.
      |                                        BIT2 (0x04) = Over current.
      | */
  (junction 10) -> (junction 14) [order 2] : {
      | trig_clear_p1504_malf ;
      | }
  (junction 10) -> (junction 11) [order 1] : /* test required */
      | [    (IAC_OT_REQ == 1)...
      | && (ccm_ena_flg == 1) ]
  (junction 11) -> (junction 12) [order 2]
  (junction 11) -> (junction 13) [order 1] : /* Freeze Timer */
      | [    ( (abv_percent <= IAC_TST_DC)...
      |  && !(abv_status & BIT3) ) ]
  (junction 12) -> (junction 13) [order 1] : [    (abv_status & BIT3 ) ...
      |   || (abv_status & BIT2 )  ]
      | {
      | trig_incr_tmr4 ;
      | }
  (junction 12) -> (junction 13) [order 2] : {
      | trig_rst_tmr4 ;
      | }
  (junction 13) -> (junction 14) [order 1] : [iac_er_tmr4 > IAC_ER_TM4]
      | {
      | trig_set_p1504_malf ;
      | }
  (junction 13) -> (junction 14) [order 2] : {
      | trig_clear_p1504_malf ;
      | }
  data: abv_percent input double size=1; abv_status input uint8 size=1; ccm_ena_flg input boolean size=1; iac_er_tmr4 input double size=1; BIT2 constant uint8 size=1 =0x04; BIT3 constant uint8 size=1 =0x08; IAC_ER_TM4 parameter double size=1; IAC_TST_DC parameter double size=1; IAC_OT_REQ parameter boolean size=1
  events: trig_incr_tmr4 output FUNCTION_CALL_EVENT; trig_rst_tmr4 output FUNCTION_CALL_EVENT; trig_set_p1504_malf output FUNCTION_CALL_EVENT; trig_clear_p1504_malf output FUNCTION_CALL_EVENT; trig_fault_code_setting input FUNCTION_CALL_EVENT

== stateflow chart mfordmodel_v1/iac_v04_001_001/iac_executive/iac_executive_ctl ==
  state iac_executive [parallel]
    settings: executionOrder=1
    iac_executive -> (junction 20)
    (default) -> (junction 20) : {
        | ml_iac_sys_mode_lst = 0;
        | ml_sys_mode_init = 0;
        | }
    (junction 20) -> (junction 21) : {
        | ml_normal_init = 2;
        | do_iac_dlt_time_calc ;
        | trig_activate_desired_rpm ;
        | trig_runup_flag_timer ;
        | trig_misc_calcs;
        | }
    (junction 21) -> (junction 27) [order 1] : /* Output override (substitute) for
        |    'flowrate' is enabled */
        | [ ( osc_ena_0 == OSC_MASK ) ...
        | && ( osc_state == 2 ) ]
    (junction 21) -> (junction 22) [order 2]
    (junction 22) -> (junction 27) [order 1] : /* Performing diagnostics */
        | [ (er_isc_hld == 1)  || ...
        |   (osm_eo_on == 1) || ...
        |   (osm_eo_off == 1) ]
    (junction 22) -> (junction 23) [order 2]
    (junction 23) -> (junction 29) [order 1] : /* Supply crank flowrate */
        | [crkflg == 1]
        | {
        | trig_crank_mode ;
        | iac_sys_mode =...
        |  IAC_SYS_MODE_CRANKING ;
        | }
    (junction 23) -> (junction 24) [order 2]
    (junction 24) -> (junction 25) [order 2]
    (junction 24) -> (junction 29) [order 1] : /* Supply failure mode flowrate */
        | [  ( mfmflg == 1 )...
        |  && ( tfmflg == 1 ) ]
        | {
        | do_failure_mode ;
        | iac_sys_mode =...
        |  IAC_SYS_MODE_FAILURE ;
        | }
    (junction 25) -> (junction 26) [order 2]
    (junction 25) -> (junction 29) [order 1] : /* Runup not yet complete
        |     continue to supply crank
        |     flowrate  */
        | [runup_flg == 0]
        | {
        | trig_crank_mode ;
        | iac_sys_mode =...
        | IAC_SYS_MODE_CRANKING;
        | }
    (junction 26) -> (junction 28) [order 1] : /* Reinit when re-entering Normal mode */
        | [ (ml_sys_mode_init == 1) ...
        |  && (ml_iac_sys_mode_lst !=...
        |     IAC_SYS_MODE_NORMAL) ]
        | {
        |  ml_normal_init = 1;
        | }
    (junction 26) -> (junction 28) [order 2]
    (junction 27) -> (junction 29) : {
        | trig_external_override_mode  ;
        | iac_sys_mode =...
        |  IAC_SYS_MODE_OUTPUT_STATE_CONTROL ;
        | }
    (junction 28) -> (junction 29) : {
        | trig_activate_normal_mode  ;
        | iac_sys_mode = IAC_SYS_MODE_NORMAL;
        | }
    (junction 29) -> (junction 30) : {
        | trig_fault_code_setting ;
        | ml_iac_sys_mode_lst = iac_sys_mode;
        | ml_sys_mode_init = 1;
        | }
  data: crkflg input boolean size=1; er_isc_hld input boolean size=1; mfmflg input boolean size=1; osc_ena_0 input uint32 size=1; osc_state input int16 size=1; osm_eo_off input boolean size=1; osm_eo_on input boolean size=1; tfmflg input boolean size=1; runup_flg input boolean size=1; OSC_MASK parameter uint8 size=1; ml_normal_init output uint8 size=1 =2; IAC_SYS_MODE_NORMAL constant uint8 size=1 =4; iac_sys_mode local uint8 size=1; IAC_SYS_MODE_OUTPUT_STATE_CONTROL constant uint8 size=1 =1; IAC_SYS_MODE_CRANKING constant uint8 size=1 =2; IAC_SYS_MODE_FAILURE constant uint8 size=1 =3; ml_iac_sys_mode_lst local uint8 size=1; ml_sys_mode_init local boolean size=1
  events: trig_activate_desired_rpm output FUNCTION_CALL_EVENT; trig_external_override_mode output FUNCTION_CALL_EVENT; trig_crank_mode output FUNCTION_CALL_EVENT; do_failure_mode output FUNCTION_CALL_EVENT; trig_runup_flag_timer output FUNCTION_CALL_EVENT; trig_activate_normal_mode output FUNCTION_CALL_EVENT; trig_fault_code_setting output FUNCTION_CALL_EVENT; trig_iac_executive input FUNCTION_CALL_EVENT; trig_misc_calcs output FUNCTION_CALL_EVENT; do_iac_dlt_time_calc output FUNCTION_CALL_EVENT

== stateflow chart mfordmodel_v1/iac_v04_001_001/iac_executive/mode_control/crank_mode/crank_mode_ctl ==
  (default) -> (junction 5) : trig_crank_mode
  (junction 5) -> (junction 6) [order 2] : {
      | ml_flow_sel_sw = 1  ;
      | }
  (junction 5) -> (junction 6) [order 1] : [tslpip >= 2.0]
      | {
      | ml_flow_sel_sw = 2 ;
      | }
  (junction 6) -> (junction 7) : {
      | do_crank_calcs ;
      | }
  data: ml_flow_sel_sw output uint8 size=1; tslpip input double size=1
  events: do_crank_calcs output FUNCTION_CALL_EVENT; trig_crank_mode input FUNCTION_CALL_EVENT

== stateflow chart mfordmodel_v1/iac_v04_001_001/iac_executive/mode_control/external_override_mode/external_override_mode_ctl ==
  (default) -> (junction 9) : trig_external_override_mode
  (junction 9) -> (junction 10) [order 2]
  (junction 9) -> (junction 12) [order 1] : /* osc_check() */
      | [   ( osc_ena_0 == OSC_MASK)...
      | && (osc_state == 2) ]
      | {
      | do_substitute;
      | ml_flow_sel_sw = 1;
      | }
  (junction 10) -> (junction 12) [order 1] : [osm_eo_on ==1]
      | {
      | ml_flow_sel_sw = 2 ;
      | }
  (junction 10) -> (junction 11) [order 2]
  (junction 11) -> (junction 12) [order 2] : {
      | ml_flow_sel_sw = 4;
      | }
  (junction 11) -> (junction 12) [order 1] : [osm_eo_off == 1]
      | {
      | ml_flow_sel_sw = 3;
      | }
  (junction 12) -> (junction 13) : {
      | do_flowrate_set;
      | }
  data: ml_flow_sel_sw output uint8 size=1; osm_eo_off input double size=1; osm_eo_on input double size=1; osc_ena_0 input double size=1; osc_state input double size=1; OSC_MASK parameter double size=1
  events: trig_external_override_mode input FUNCTION_CALL_EVENT; do_flowrate_set output FUNCTION_CALL_EVENT; do_substitute output FUNCTION_CALL_EVENT

== stateflow chart mfordmodel_v1/iac_v04_001_001/iac_executive/fault_code_setting/type1_fault_code/fault code_ctl ==
  state clear [parallel]
    settings: executionOrder=1
    clear -> (junction 9) : clear_malf
    (default) -> (junction 9) : clear_malf
    (junction 9) -> (junction 12) : {pxxxmalf = 0;}
  state malf [parallel]
    settings: executionOrder=2
    malf -> (junction 10) : malfunction
    (default) -> (junction 10) : malfunction
    (junction 10) -> (junction 11) : {pxxxmalf = 1;}
  data: pxxxmalf output double
  events: malfunction input FUNCTION_CALL_EVENT; clear_malf input FUNCTION_CALL_EVENT

== stateflow chart mfordmodel_v1/iac_v04_001_001/iac_executive/runup_flag_timer/runup_flag_timer_ctl ==
  state select_runup_mode [parallel]
    settings: executionOrder=1
    (default) -> (junction 17)
    (junction 17) -> (junction 18) [order 2] : {
        | pre_runup_tmp = RUNUP_DIFF ;
        | }
    (junction 17) -> (junction 18) [order 1] : [alt_cal_flg == 1]
        | {
        | pre_runup_tmp = RUNUP_DIFF_A ;
        | }
  state runup_check [parallel]
    settings: executionOrder=2
    state runup_not_complete
      runup_not_complete -> (junction 19) [order 1]
      (default) -> (junction 19)
      (junction 19) -> (junction 21) : {
          | runup_flg = 0 ;
          | trig_rst_runup_tmr  ;
          | }
    state runup_complete
      runup_complete -> (junction 20) [order 1]
      (default) -> (junction 20)
      (junction 20) -> (junction 22) : {
          | runup_flg = 1 ;
          | trig_incr_runup_tmr;
          | }
    (default) -> runup_not_complete
    runup_complete -> runup_not_complete [order 1] : [eng_stalled == 1]
    runup_not_complete -> runup_complete [order 1] : [ (eng_stalled == 0)...
        |  && (engine_speed > (dsdrpm + pre_runup_tmp)) ]
  data: dsdrpm input double size=1; alt_cal_flg input boolean size=1; runup_flg output boolean size=1; eng_stalled input boolean size=1; engine_speed input double size=1; pre_runup_tmp local double size=1; RUNUP_DIFF_A parameter double size=1; RUNUP_DIFF parameter double size=1
  events: trig_incr_runup_tmr output FUNCTION_CALL_EVENT; trig_rst_runup_tmr output FUNCTION_CALL_EVENT; trig_runup_flag_timer input FUNCTION_CALL_EVENT

== stateflow chart mfordmodel_v1/iac_v04_001_001/activate_desired_rpm/hicam_rpm_request/hicam_rpm_request_ctl ==
  (default) -> (junction 35) : trig_hicam_rpm_request
      | { isadd_buzz_tmp = 0.0;
      |   isadd_st_ect_tmp = 0.0;
      |   isadd_st_act_tmp = 0.0;
      |   isadd_ect_tmp = 0.0;
      |   do_fox_calcs;
      |   hicam_source = ( hicam_source & HICAM_SOURCE_CMD_EXT); }
  (junction 42) -> (junction 34) : /* Connector */
  (junction 34) -> (junction 37) [order 2] : { flg_st_act = 1; }
  (junction 34) -> (junction 37) [order 1] : [ ( flg_st_act == 0 )...
      |  && (atmr1 < TKDTN )...
      |  && (ml_ctrl_flg == 1) ]
      | { isadd_st_act_tmp = ml_fn826b;
      |   hicam_source |=...
      |   HICAM_SOURCE_ACT_AND_THROTTLE_DEPENDENT; }
  (junction 35) -> (junction 36) [order 2] : { pre_bzztm_tmp = BZZTM;
      |   pre_bzzrpm_tmp = BZZRPM; }
  (junction 35) -> (junction 36) [order 1] : [ alt_cal_flg == 1]
      | { pre_bzztm_tmp = BZZTM_ALT;
      |   pre_bzzrpm_tmp =BZZRPM_ALT; }
  (junction 36) -> (junction 38) [order 2]
  (junction 36) -> (junction 38) [order 1] : [ atmr1 < pre_bzztm_tmp ]
      | { isadd_buzz_tmp = pre_bzzrpm_tmp;
      |   hicam_source |= HICAM_SOURCE_SINCE_LEAVING_CRANK; }
  (junction 37) -> (junction 39) [order 1] : [ dndsup == 1 ]
      | { isadd_act_tmp = ml_isadd_min;
      |   hicam_source |=...
      |   HICAM_SOURCE_ACT; }
  (junction 37) -> (junction 39) [order 2] : { isadd_act_tmp = ml_fn825b; }
  (junction 38) -> (junction 40) [order 1] : [   (apt != CLOSED_THROTTLE)...
      |  && (iac_apt_lst == CLOSED_THROTTLE) ]
      | { ctptfg = 1; }
  (junction 38) -> (junction 40) [order 2] : { ctptfg = 0; }
  (junction 39) -> (junction 41) [order 1] : [ alt_cal_flg == 1 ]
      | { isadd_ect_tmp = ml_fn825a_alt; }
  (junction 39) -> (junction 41) [order 2] : { isadd_ect_tmp = ml_fn825a; }
  (junction 40) -> (junction 43) [order 2] : { ptctfg = 0; }
  (junction 40) -> (junction 43) [order 1] : [   (apt == CLOSED_THROTTLE)...
      |  && (iac_apt_lst != CLOSED_THROTTLE) ]
      | { ptctfg = 1; }
  (junction 41) -> (junction 44) [order 2]
  (junction 41) -> (junction 44) [order 1] : [ isadd_ect_tmp > 0.0 ]
      | { hicam_source |=...
      |   HICAM_SOURCE_ECT; }
  (junction 53) -> (junction 42)
  (junction 43) -> (junction 45) : { iac_apt_lst = apt; }
  (junction 44) -> (junction 46) [order 1] : [ ext_cmd < CMD_LITOFF ]
  (junction 44) -> (junction 47) [order 2]
  (junction 45) -> (junction 48) [order 2] : { ml_ctrl_flg = 0; }
  (junction 45) -> (junction 48) [order 1] : [  ( ctptfg == 0)...
      |  || ( crkflg == 1)...
      |  || ( isadd_buzz_tmp != 0.0) ]
      | { ml_ctrl_flg = 1; }
  (junction 46) -> (junction 49) [order 1] : [ runup_flg == 0 ]
      | {ml_isadd_sw = 1;}
  (junction 46) -> (junction 49) [order 2] : { ml_ramp_sw = 1;
      |  ml_isadd_sw = 2;
      |  do_isadd_ramp; }
  (junction 47) -> (junction 51) [order 2] : { ml_isadd_sw = 3; }
  (junction 47) -> (junction 51) [order 1] : [ ext_cmd > CMD_STABLE ]
      | { ml_isadd_sw = 2;
      |   ml_ramp_sw = 2;
      |   do_isadd_ramp;
      |   hicam_source &=...
      |   ~HICAM_SOURCE_CMD_EXT; }
  (junction 48) -> (junction 53) [order 2] : { flg_st_ect = 1; }
  (junction 48) -> (junction 50) [order 1] : [ ( flg_st_ect == 0 )...
      |  && ( atmr1 < ml_fn803a )...
      |  && (ml_ctrl_flg == 1) ]
  (junction 49) -> (junction 51) : {  hicam_source |=...
      |   HICAM_SOURCE_CMD_EXT; }
  (junction 50) -> (junction 53) : [ (AUTO_TRNS_SW == 0 )...
      |  || ( ndsflg == 0 ) ]
      | { isadd_st_ect_tmp = ml_fn826a;
      |   hicam_source |=...
      |   HICAM_SOURCE_ECT_AT_START_AND_THROTTLE_DEPENDENT; }
  (junction 51) -> (junction 52) : { do_hicam_calc; }
  data: isadd_act_tmp output double size=1; isadd_ect_tmp output double size=1; isadd_st_ect_tmp output double size=1; isadd_st_act_tmp output double size=1; isadd_buzz_tmp output double size=1; ml_isadd_sw output uint8 size=1 =4; alt_cal_flg input boolean size=1; atmr1 input double size=1; apt input double size=1; crkflg input boolean size=1; ndsflg input boolean size=1; dndsup input boolean size=1; ext_cmd input double size=1; runup_flg input boolean size=1; ml_isadd_min input double size=1; ml_fn825a_alt input double size=1; ml_fn825a input double size=1; ml_fn826b input double size=1; ml_fn826a input double size=1; ml_fn803a input double size=1; ml_fn825b input double size=1; pre_bzzrpm_tmp local double size=1; ml_ramp_sw output uint8 size=1; ctptfg output boolean size=1; ptctfg output boolean size=1; iac_apt_lst local int8 size=1; CMD_LITOFF parameter double size=1; CMD_STABLE parameter double size=1; AUTO_TRNS_SW parameter uint8 size=1; flg_st_act local boolean size=1; flg_st_ect local boolean size=1; CLOSED_THROTTLE constant int8 size=1 =-1; HCAM_ACT_CLP parameter double size=1; HICAM_SOURCE_ACT constant uint8 size=1 =8; HICAM_SOURCE_ACT_AND_THROTTLE_DEPENDENT constant uint8 size=1 =4; HICAM_SOURCE_CMD_EXT constant uint8 size=1 =32; HICAM_SOURCE_ECT constant uint8 size=1 =16; HICAM_SOURCE_ECT_AT_START_AND_THROTTLE_DEPENDENT constant uint8 size=1 =2; HICAM_SOURCE_SINCE_LEAVING_CRANK constant uint8 size=1 =1; BZZTM parameter double size=1; BZZRPM parameter double size=1; BZZTM_ALT parameter double size=1; TKDTN parameter double size=1; BZZRPM_ALT parameter double size=1; pre_bzztm_tmp local double size=1; ml_ctrl_flg local uint8 size=1; hicam_source local uint8 size=1
  events: trig_hicam_rpm_request input FUNCTION_CALL_EVENT; do_hicam_calc output FUNCTION_CALL_EVENT; do_isadd_ramp output FUNCTION_CALL_EVENT; do_fox_calcs output FUNCTION_CALL_EVENT
